simulink model "testDataLoggerLocal"  (R2014a)
settings: Solver=FixedStepDiscrete  StartTime=0.0  StopTime=Inf  FixedStep=0.001  RelTol=1e-3
PreLoadFcn:
  | testDataLoggerLocal_Initialize();
InitFcn:
  | testDataLoggerLocal_Initialize();
undefined symbols (not defined in the file or in its folder): fn2, libBusSerialize
libraries: simulink x4, libButtons x3, dspnetwork x3
settings Model: xpc_rtwmakecfg_data=_xpcnblib__xpcetherlib__xpcether8255xlib__xpcetherGbElib_  BufferReuse=off  Creator=shenoylab  LastModifiedBy=shenoylab
settings SolverCC: EnableConcurrentExecution=on
settings DataIOCC: SignalLoggingSaveFormat=ModelDataLogs
settings OptimizationCC: BlockReduction=off  OptimizeBlockIOStorage=off  BufferReuse=off  GlobalBufferReuse=off  ExpressionFolding=off  LocalBlockOutputs=off
settings DebuggingCC: SaveWithDisabledLinksMsg=none  MultiTaskDSMMsg=warning  MultiTaskCondExecSysMsg=none  StateNameClashWarn=warning
settings HardwareCC: ProdIntDivRoundTo=Zero  ProdEndianess=LittleEndian  ProdHWDeviceType=Generic->32-bit x86 compatible
settings RTWCC: SystemTargetFile=slrt.tlc  TemplateMakefile=slrt_default_tmf  Description=Simulink Real-Time  GenerateReport=on  ProcessScript=slrt_make_rtw_hook  LaunchReport=on  IncludeERTFirstTime=on  RTWCompilerOptimization=On
settings CodeAppCC: MATLABSourceComments=on
settings TargetCC: CodeReplacementLibrary=XPC_BLAS  ParMdlRefBuildCompliant=on  ConcurrentExecutionCompliant=on  MatFileLogging=on  EnableShiftOperators=on  MATLABClassNameForMDSCustomization=xpcAperiodicCustomization

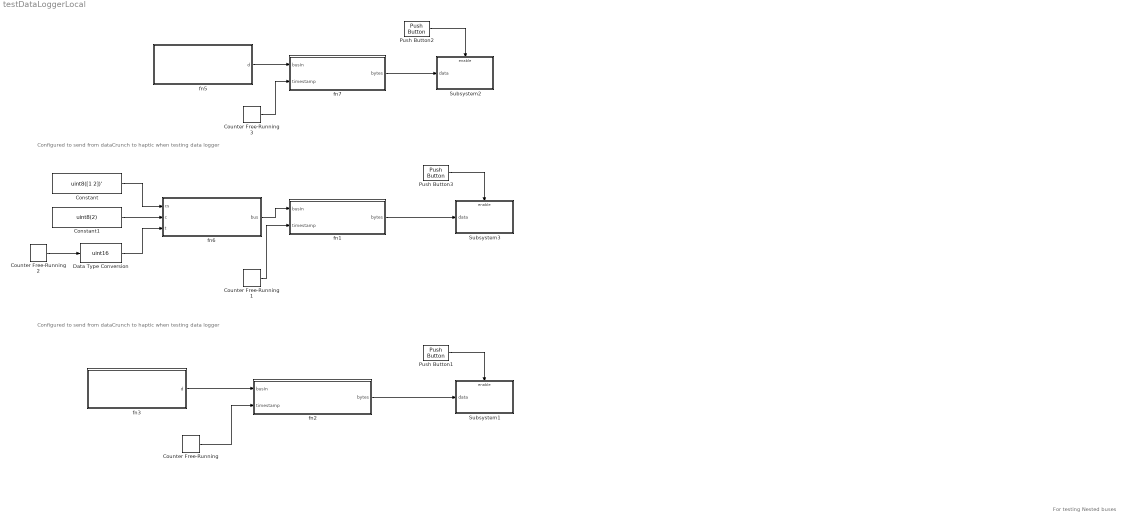
== system testDataLoggerLocal ==
  note: Configured to send from dataCrunch to haptic when testing data logger
  note: For testing Nested buses
  note: Configured to send from dataCrunch to haptic when testing data logger
  Constant : Constant  Value=uint8([1 2])'
  Constant1 : Constant  Value=uint8(2)
  Counter Free-Running : simulink/Sources/Counter Free-Running  NumBits=32  tsamp=-1
  Counter Free-Running1 : simulink/Sources/Counter Free-Running  NumBits=32  tsamp=-1
  Counter Free-Running2 : simulink/Sources/Counter Free-Running  NumBits=16  tsamp=-1
  Counter Free-Running3 : simulink/Sources/Counter Free-Running  NumBits=32  tsamp=-1
  Data Type Conversion : DataTypeConversion  OutDataTypeStr=uint16
  Push Button1 : libButtons/Push Button  Ts=0.001
  Push Button2 : libButtons/Push Button  Ts=0.001
  Push Button3 : libButtons/Push Button  Ts=0.001
  Subsystem1 : Subsystem
  Subsystem2 : Subsystem
  Subsystem3 : Subsystem
  fn1 : MATLAB Function  AncestorBlock=libBusSerialize/fn2  TreatAsAtomicUnit=on  mask(BusSerialize: serialize block){busType=Bus: TestBusOuter, groupType=Parameters, groupName='testBusOuter'}
      mask prompts: busType "Bus Type"; groupType "Group Type"; groupName "Group Name"
      mask help: Select the bus type below to serialize.
      mask init:
      | BusSerialize.maskSerializeWithDataLoggerHeaderBlockUpdate(gcb)
  fn2 : MATLAB Function  AncestorBlock=libBusSerialize/fn2  TreatAsAtomicUnit=on  mask(BusSerialize: serialize block){busType=Bus: DataLoggerControlBus, groupType=Control, groupName='control'}
      mask prompts: busType "Bus Type"; groupType "Group Type"; groupName "Group Name"
      mask help: Select the bus type below to serialize.
      mask init:
      | BusSerialize.maskSerializeWithDataLoggerHeaderBlockUpdate(gcb)
  fn3 : MATLAB Function  TreatAsAtomicUnit=on
  fn5 : MATLAB Function  TreatAsAtomicUnit=on
  fn6 : MATLAB Function  TreatAsAtomicUnit=on
  fn7 : MATLAB Function  AncestorBlock=libBusSerialize/fn2  TreatAsAtomicUnit=on  mask(BusSerialize: serialize block){busType=Bus: TestBus, groupType=Analog Channels, groupName='analog'}
      mask prompts: busType "Bus Type"; groupType "Group Type"; groupName "Group Name"
      mask help: Select the bus type below to serialize.
      mask init:
      | BusSerialize.maskSerializeWithDataLoggerHeaderBlockUpdate(gcb)
  wires:
  fn6/1(bus) -> fn1/1(busIn)
  Constant/1 -> fn6/1(cs)
  Constant1/1 -> fn6/2(c)
  Data Type Conversion/1 -> fn6/3(t)
  Counter Free-Running2/1 -> Data Type Conversion/1
  fn3/1(d) -> fn2/1(busIn)
  Counter Free-Running/1 -> fn2/2(timestamp)
  Counter Free-Running1/1 -> fn1/2(timestamp)
  fn7/1(bytes) -> Subsystem2/1(data)
  Push Button2/1 -> Subsystem2/Enable
  fn5/1(d) -> fn7/1(busIn)
  Counter Free-Running3/1 -> fn7/2(timestamp)
  Push Button3/1 -> Subsystem3/Enable
  fn1/1(bytes) -> Subsystem3/1(data)
  fn2/1(bytes) -> Subsystem1/1(data)
  Push Button1/1 -> Subsystem1/Enable

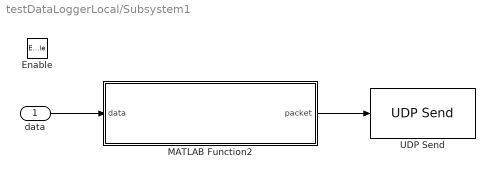
== system testDataLoggerLocal/Subsystem1 ==
  data : Inport
  Enable : EnablePort  PropagateVarSize=During execution
  MATLAB Function2 : MATLAB Function  TreatAsAtomicUnit=on
  UDP Send : dspnetwork/UDP Send  remoteURL='192.168.1.255'  remotePort=29000  localURL='0.0.0.0'  localPortSource=Automatically determine  localPort=10000  sampletime=-1  separateLengthPort=0
  wires:
  data/1 -> MATLAB Function2/1(data)
  MATLAB Function2/1(packet) -> UDP Send/1

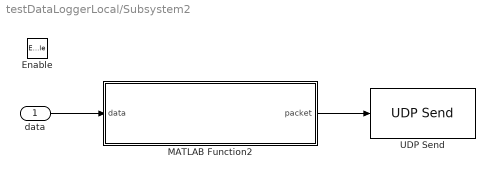
== system testDataLoggerLocal/Subsystem2 ==
  data : Inport
  Enable : EnablePort  PropagateVarSize=During execution
  MATLAB Function2 : MATLAB Function  TreatAsAtomicUnit=on
  UDP Send : dspnetwork/UDP Send  remoteURL='192.168.1.255'  remotePort=29000  localURL='0.0.0.0'  localPortSource=Automatically determine  localPort=10000  sampletime=-1  separateLengthPort=0
  wires:
  data/1 -> MATLAB Function2/1(data)
  MATLAB Function2/1(packet) -> UDP Send/1

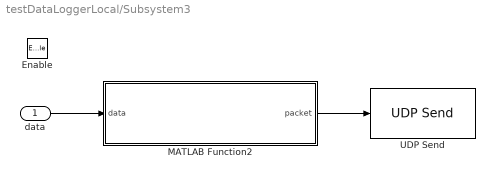
== system testDataLoggerLocal/Subsystem3 ==
  data : Inport
  Enable : EnablePort  PropagateVarSize=During execution
  MATLAB Function2 : MATLAB Function  TreatAsAtomicUnit=on
  UDP Send : dspnetwork/UDP Send  remoteURL='192.168.1.255'  remotePort=29000  localURL='0.0.0.0'  localPortSource=Automatically determine  localPort=10000  sampletime=-1  separateLengthPort=0
  wires:
  data/1 -> MATLAB Function2/1(data)
  MATLAB Function2/1(packet) -> UDP Send/1

== matlab function testDataLoggerLocal/fn1 ==
  data: busIn input Bus: TestBusOuter size=1; bytes output uint8 size=154; timestamp input uint32 size=1
function bytes = dataLoggerSerialize(busIn, timestamp)
%#codegen
    bytes = testDataLoggerLocalLib.serializeBusWithDataLoggerHeader_TestBusOuter(busIn, uint8(2), uint8('testBusOuter'), timestamp);
end

== matlab function testDataLoggerLocal/Subsystem1/MATLAB Function2 ==
  data: data input uint8; packet output uint8 size=65000
function packet = prependLengthChecksumHeader(data)
%#codegen

% 8 byte header on first packet containing '#udp', 2 byte length, 2 byte checksum

coder.varsize('packet', 65000);

% include custom 8 byte custom header with length and checksum
headerPre = zeros(4, 1, 'uint8');
headerPre(1:2) = typecast(uint16(numel(data)), 'uint8');
checksum = uint16(mod(sum(uint32(data)), uint32(65536)));
headerPre(3:4) = typecast(checksum, 'uint8');
packet = [headerPre; data];

== matlab function testDataLoggerLocal/Subsystem3/MATLAB Function2 ==
  data: data input uint8; packet output uint8 size=65000
function packet = prependLengthChecksumHeader(data)
%#codegen

% 8 byte header on first packet containing '#udp', 2 byte length, 2 byte checksum

coder.varsize('packet', 65000);

% include custom 8 byte custom header with length and checksum
headerPre = zeros(4, 1, 'uint8');
headerPre(1:2) = typecast(uint16(numel(data)), 'uint8');
checksum = uint16(mod(sum(uint32(data)), uint32(65536)));
headerPre(3:4) = typecast(checksum, 'uint8');
packet = [headerPre; data];

== matlab function testDataLoggerLocal/fn2 ==
  data: busIn input Bus: DataLoggerControlBus size=1; bytes output uint8 size=253; timestamp input uint32 size=1
function bytes = dataLoggerSerialize(busIn, timestamp)
%#codegen
    bytes = testDataLoggerLocalLib.serializeBusWithDataLoggerHeader_DataLoggerControlBus(busIn, uint8(1), uint8('control'), timestamp);
end

== matlab function testDataLoggerLocal/fn3 ==
  data: d output Bus: DataLoggerControlBus size=1
function d = createBus()

d.dataStore = uint8('testStore')';
d.subject = uint8('testSubj')';
d.protocol =  uint8('testProto')';
d.protocolVersion = uint32(20140428);
d.saveTag = uint32(1);
d.nextTrial = uint8(1);

== matlab function testDataLoggerLocal/fn6 ==
  data: bus output Bus: TestBusOuter size=1; cs input uint8; c input uint8; t input uint16
function bus = createBus(cs, c, t)

P1.centerSize = uint8(cs);
P1.holdWindowCenter = uint8(c);
P1.holdWindowTarget = uint16(t);

bus.val1 = uint8(3);
bus.val2 = uint8('hello')';
bus.nested = P1;

== matlab function testDataLoggerLocal/fn5 ==
  data: d output Bus: TestBus size=1
function d = createBus()

d.centerSize = ones(255, 20, 'uint8');
d.holdWindowCenter = uint8(15);
d.holdWindowTarget = uint8('helloWorld')';

== matlab function testDataLoggerLocal/Subsystem2/MATLAB Function2 ==
  data: data input uint8; packet output uint8 size=65000
function packet = prependLengthChecksumHeader(data)
%#codegen

% 8 byte header on first packet containing '#udp', 2 byte length, 2 byte checksum

coder.varsize('packet', 65000);

% include custom 8 byte custom header with length and checksum
headerPre = zeros(4, 1, 'uint8');
headerPre(1:2) = typecast(uint16(numel(data)), 'uint8');
checksum = uint16(mod(sum(uint32(data)), uint32(65536)));
headerPre(3:4) = typecast(checksum, 'uint8');
packet = [headerPre; data];

== matlab function testDataLoggerLocal/fn7 ==
  data: busIn input Bus: TestBus size=1; bytes output uint8 size=6511; timestamp input uint32 size=1
function bytes = dataLoggerSerialize(busIn, timestamp)
%#codegen
    bytes = testDataLoggerLocalLib.serializeBusWithDataLoggerHeader_TestBus(busIn, uint8(3), uint8('analog'), timestamp);
end
